simulink model "glucose_type2"  (R2020b)
settings: Solver=VariableStepAuto  StartTime=0.0  StopTime=20.0  RelTol=1e-3
settings Model: Creator=duzun  LastModifiedBy=duzun

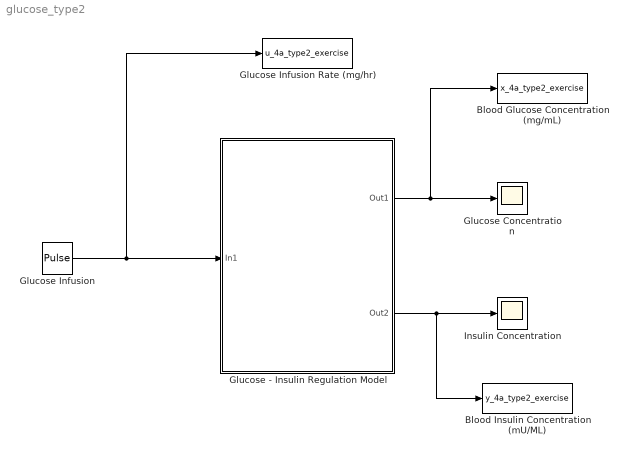
== system glucose_type2 ==
  Blood Glucose Concentration (mg/mL) : ToWorkspace  VariableName=x_4a_type2_exercise  SaveFormat=Timeseries  SampleTime=-1
  Blood Insulin Concentration (mU/ML) : ToWorkspace  VariableName=y_4a_type2_exercise  SaveFormat=Timeseries  SampleTime=-1
  Glucose - Insulin Regulation Model : Subsystem
  Glucose Concentration : Scope
  Glucose Infusion : DiscretePulseGenerator  PulseType=Time based  Amplitude=100000  Period=5  PulseWidth=5  PhaseDelay=0.5
  Glucose Infusion Rate (mg/hr) : ToWorkspace  VariableName=u_4a_type2_exercise  SaveFormat=Timeseries  SampleTime=-1
  Insulin Concentration : Scope
  wires:
  Glucose - Insulin Regulation Model/2(Out2) -> Blood Insulin Concentration (mU/ML)/1, Insulin Concentration/1
  Glucose Infusion/1 -> Glucose Infusion Rate (mg/hr)/1, Glucose - Insulin Regulation Model/1(In1)
  Glucose - Insulin Regulation Model/1(Out1) -> Blood Glucose Concentration (mg/mL)/1, Glucose Concentration/1

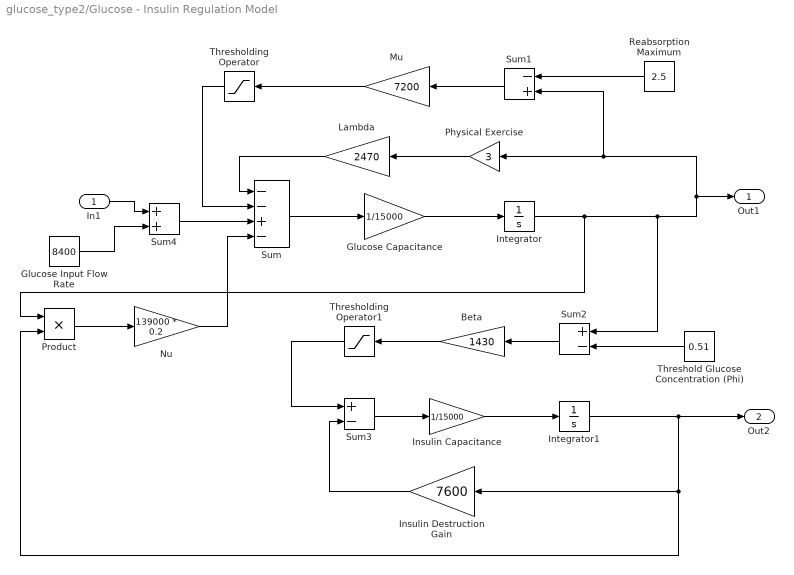
== system glucose_type2/Glucose - Insulin Regulation Model ==
  In1 : Inport
  Beta : Gain  Gain=1430
  Glucose Capacitance : Gain  Gain=1/15000
  Glucose Input Flow Rate : Constant  Value=8400
  Insulin Capacitance : Gain  Gain=1/15000
  Insulin Destruction Gain : Gain  Gain=7600
  Integrator : Integrator  InitialCondition=0.81
  Integrator1 : Integrator  InitialCondition=0.055
  Lambda : Gain  Gain=2470
  Mu : Gain  Gain=7200
  Nu : Gain  Gain=139000 * 0.2
  Physical Exercise : Gain  Gain=3
  Product : Product
  Reabsorption Maximum : Constant  Value=2.5
  Sum : Sum  Inputs=--+-
  Sum1 : Sum  Inputs=-+
  Sum2 : Sum  Inputs=+-
  Sum3 : Sum  Inputs=+-
  Sum4 : Sum
  Threshold Glucose Concentration (Phi) : Constant  Value=0.51
  Thresholding Operator : Saturate  UpperLimit=100000  LowerLimit=0
  Thresholding Operator1 : Saturate  UpperLimit=10000  LowerLimit=0
  Out1 : Outport
  Out2 : Outport  Port=2
  wires:
  In1/1 -> Sum4/1
  Glucose Input Flow Rate/1 -> Sum4/2
  Sum4/1 -> Sum/3
  Sum/1 -> Glucose Capacitance/1
  Glucose Capacitance/1 -> Integrator/1
  Integrator/1 -> Product/1, Sum2/1, Sum1/2, Physical Exercise/1, Out1/1
  Product/1 -> Nu/1
  Sum1/1 -> Mu/1
  Reabsorption Maximum/1 -> Sum1/1
  Mu/1 -> Thresholding Operator/1
  Thresholding Operator/1 -> Sum/2
  Lambda/1 -> Sum/1
  Nu/1 -> Sum/4
  Beta/1 -> Thresholding Operator1/1
  Sum2/1 -> Beta/1
  Threshold Glucose Concentration (Phi)/1 -> Sum2/2
  Thresholding Operator1/1 -> Sum3/1
  Insulin Destruction Gain/1 -> Sum3/2
  Sum3/1 -> Insulin Capacitance/1
  Insulin Capacitance/1 -> Integrator1/1
  Integrator1/1 -> Insulin Destruction Gain/1, Product/2, Out2/1
  Physical Exercise/1 -> Lambda/1
